simulink model "lb1"  (R2023b)
settings: Solver=VariableStepAuto  StartTime=0.0  StopTime=10.0  RelTol=1e-3
values from neighbouring files (symbols this model uses):
  A = [ ... (first row only)    [lw1_params.m]
  B = [ 0 ; 0 ; -a_3+a_5*a_11 ; -a_5 ]    [lw1_params.m]
  G = [ 1 ; 0 ; 0 ; 0 ]    [lw1_params.m]
  myConstant = 1    [lw1_2.m]
settings Model: Creator=kek  LastModifiedBy=kek

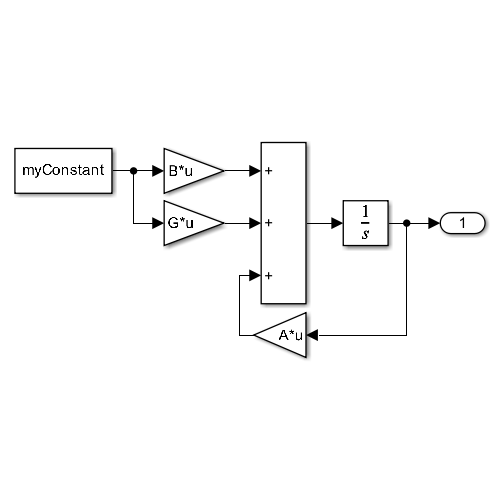
[thumbnail: Simulink's stored preview of the top-level diagram]
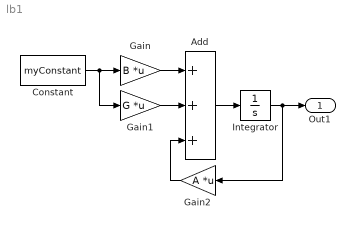
== system lb1 ==
  Add : Sum  Inputs=+++
  Constant : Constant  Value=myConstant
  Gain : Gain  Gain=B  Multiplication=Matrix(K*u)
  Gain1 : Gain  Gain=G  Multiplication=Matrix(K*u)
  Gain2 : Gain  Gain=A  Multiplication=Matrix(K*u)
  Integrator : Integrator
  Out1 : Outport
  wires:
  Constant/1 -> Gain1/1, Gain/1
  Gain/1 -> Add/1
  Gain1/1 -> Add/2
  Gain2/1 -> Add/3
  Add/1 -> Integrator/1
  Integrator/1 -> Out1/1, Gain2/1
